simulink model "V3ASM"  (R2020b)
(part 2 of 23)

  Revolute39 : sm_lib/Joints/Revolute Joint  JointMode=Normal  SenseConstraintForce=off  SenseConstraintForceX=off  SenseConstraintForceY=off  SenseConstraintForceZ=off  SenseConstraintTorque=off  SenseConstraintTorqueX=off  SenseConstraintTorqueY=off  SenseConstraintTorqueZ=off  SenseTotalForce=off  SenseTotalForceX=off  SenseTotalForceY=off  SenseTotalForceZ=off  SenseTotalTorque=off  SenseTotalTorqueX=off  SenseTotalTorqueY=off  SenseTotalTorqueZ=off  CompositeWrenchDir=FollowerOnBase  CompositeWrenchFrame=BaseFrame  EquilibriumPosition=0  EquilibriumPositionUnits=deg  SpringStiffness=0  SpringStiffnessUnits=N*m/deg  DampingCoefficient=0  DampingCoefficientUnits=N*m/(deg/s)  TorqueActuationMode=NoTorque  MotionActuationMode=ComputedMotion  SensePosition=off  SenseVelocity=off  SenseAcceleration=off  SenseTorqueForce=off  SenseLowerLimitTorqueForce=off  SenseUpperLimitTorqueForce=off  LowerLimitSpecify=off  LowerLimitBound=-90  LowerLimitBoundUnits=deg  LowerLimitStiffness=1e4  LowerLimitStiffnessUnits=N*m/deg  LowerLimitDamping=10  LowerLimitDampingUnits=N*m/(deg/s)  LowerLimitTransitionRegionWidth=0.1  LowerLimitTransitionRegionWidthUnits=deg  UpperLimitSpecify=off  UpperLimitBound=90  UpperLimitBoundUnits=deg  UpperLimitStiffness=1e4  UpperLimitStiffnessUnits=N*m/deg  UpperLimitDamping=10  UpperLimitDampingUnits=N*m/(deg/s)  UpperLimitTransitionRegionWidth=0.1  UpperLimitTransitionRegionWidthUnits=deg  PositionTargetSpecify=on  PositionTargetPriority=Low  PositionTargetValue=smiData.RevoluteJoint(40).Rz.Pos  PositionTargetValueUnits=deg  VelocityTargetSpecify=off  VelocityTargetPriority=High  VelocityTargetValue=0  VelocityTargetValueUnits=deg/s
  Revolute4 : sm_lib/Joints/Revolute Joint  JointMode=Normal  SenseConstraintForce=off  SenseConstraintForceX=off  SenseConstraintForceY=off  SenseConstraintForceZ=off  SenseConstraintTorque=off  SenseConstraintTorqueX=off  SenseConstraintTorqueY=off  SenseConstraintTorqueZ=off  SenseTotalForce=off  SenseTotalForceX=off  SenseTotalForceY=off  SenseTotalForceZ=off  SenseTotalTorque=off  SenseTotalTorqueX=off  SenseTotalTorqueY=off  SenseTotalTorqueZ=off  CompositeWrenchDir=FollowerOnBase  CompositeWrenchFrame=BaseFrame  EquilibriumPosition=0  EquilibriumPositionUnits=deg  SpringStiffness=0  SpringStiffnessUnits=N*m/deg  DampingCoefficient=0  DampingCoefficientUnits=N*m/(deg/s)  TorqueActuationMode=NoTorque  MotionActuationMode=ComputedMotion  SensePosition=off  SenseVelocity=off  SenseAcceleration=off  SenseTorqueForce=off  SenseLowerLimitTorqueForce=off  SenseUpperLimitTorqueForce=off  LowerLimitSpecify=off  LowerLimitBound=-90  LowerLimitBoundUnits=deg  LowerLimitStiffness=1e4  LowerLimitStiffnessUnits=N*m/deg  LowerLimitDamping=10  LowerLimitDampingUnits=N*m/(deg/s)  LowerLimitTransitionRegionWidth=0.1  LowerLimitTransitionRegionWidthUnits=deg  UpperLimitSpecify=off  UpperLimitBound=90  UpperLimitBoundUnits=deg  UpperLimitStiffness=1e4  UpperLimitStiffnessUnits=N*m/deg  UpperLimitDamping=10  UpperLimitDampingUnits=N*m/(deg/s)  UpperLimitTransitionRegionWidth=0.1  UpperLimitTransitionRegionWidthUnits=deg  PositionTargetSpecify=on  PositionTargetPriority=Low  PositionTargetValue=smiData.RevoluteJoint(5).Rz.Pos  PositionTargetValueUnits=deg  VelocityTargetSpecify=off  VelocityTargetPriority=High  VelocityTargetValue=0  VelocityTargetValueUnits=deg/s
  Revolute40 : sm_lib/Joints/Revolute Joint  JointMode=Normal  SenseConstraintForce=off  SenseConstraintForceX=off  SenseConstraintForceY=off  SenseConstraintForceZ=off  SenseConstraintTorque=off  SenseConstraintTorqueX=off  SenseConstraintTorqueY=off  SenseConstraintTorqueZ=off  SenseTotalForce=off  SenseTotalForceX=off  SenseTotalForceY=off  SenseTotalForceZ=off  SenseTotalTorque=off  SenseTotalTorqueX=off  SenseTotalTorqueY=off  SenseTotalTorqueZ=off  CompositeWrenchDir=FollowerOnBase  CompositeWrenchFrame=BaseFrame  EquilibriumPosition=0  EquilibriumPositionUnits=deg  SpringStiffness=0  SpringStiffnessUnits=N*m/deg  DampingCoefficient=0  DampingCoefficientUnits=N*m/(deg/s)  TorqueActuationMode=NoTorque  MotionActuationMode=ComputedMotion  SensePosition=off  SenseVelocity=off  SenseAcceleration=off  SenseTorqueForce=off  SenseLowerLimitTorqueForce=off  SenseUpperLimitTorqueForce=off  LowerLimitSpecify=off  LowerLimitBound=-90  LowerLimitBoundUnits=deg  LowerLimitStiffness=1e4  LowerLimitStiffnessUnits=N*m/deg  LowerLimitDamping=10  LowerLimitDampingUnits=N*m/(deg/s)  LowerLimitTransitionRegionWidth=0.1  LowerLimitTransitionRegionWidthUnits=deg  UpperLimitSpecify=off  UpperLimitBound=90  UpperLimitBoundUnits=deg  UpperLimitStiffness=1e4  UpperLimitStiffnessUnits=N*m/deg  UpperLimitDamping=10  UpperLimitDampingUnits=N*m/(deg/s)  UpperLimitTransitionRegionWidth=0.1  UpperLimitTransitionRegionWidthUnits=deg  PositionTargetSpecify=on  PositionTargetPriority=Low  PositionTargetValue=smiData.RevoluteJoint(41).Rz.Pos  PositionTargetValueUnits=deg  VelocityTargetSpecify=off  VelocityTargetPriority=High  VelocityTargetValue=0  VelocityTargetValueUnits=deg/s
  Revolute41 : sm_lib/Joints/Revolute Joint  JointMode=Normal  SenseConstraintForce=off  SenseConstraintForceX=off  SenseConstraintForceY=off  SenseConstraintForceZ=off  SenseConstraintTorque=off  SenseConstraintTorqueX=off  SenseConstraintTorqueY=off  SenseConstraintTorqueZ=off  SenseTotalForce=off  SenseTotalForceX=off  SenseTotalForceY=off  SenseTotalForceZ=off  SenseTotalTorque=off  SenseTotalTorqueX=off  SenseTotalTorqueY=off  SenseTotalTorqueZ=off  CompositeWrenchDir=FollowerOnBase  CompositeWrenchFrame=BaseFrame  EquilibriumPosition=0  EquilibriumPositionUnits=deg  SpringStiffness=0  SpringStiffnessUnits=N*m/deg  DampingCoefficient=0  DampingCoefficientUnits=N*m/(deg/s)  TorqueActuationMode=NoTorque  MotionActuationMode=ComputedMotion  SensePosition=off  SenseVelocity=off  SenseAcceleration=off  SenseTorqueForce=off  SenseLowerLimitTorqueForce=off  SenseUpperLimitTorqueForce=off  LowerLimitSpecify=off  LowerLimitBound=-90  LowerLimitBoundUnits=deg  LowerLimitStiffness=1e4  LowerLimitStiffnessUnits=N*m/deg  LowerLimitDamping=10  LowerLimitDampingUnits=N*m/(deg/s)  LowerLimitTransitionRegionWidth=0.1  LowerLimitTransitionRegionWidthUnits=deg  UpperLimitSpecify=off  UpperLimitBound=90  UpperLimitBoundUnits=deg  UpperLimitStiffness=1e4  UpperLimitStiffnessUnits=N*m/deg  UpperLimitDamping=10  UpperLimitDampingUnits=N*m/(deg/s)  UpperLimitTransitionRegionWidth=0.1  UpperLimitTransitionRegionWidthUnits=deg  PositionTargetSpecify=on  PositionTargetPriority=Low  PositionTargetValue=smiData.RevoluteJoint(42).Rz.Pos  PositionTargetValueUnits=deg  VelocityTargetSpecify=off  VelocityTargetPriority=High  VelocityTargetValue=0  VelocityTargetValueUnits=deg/s
  Revolute5 : sm_lib/Joints/Revolute Joint  JointMode=Normal  SenseConstraintForce=off  SenseConstraintForceX=off  SenseConstraintForceY=off  SenseConstraintForceZ=off  SenseConstraintTorque=off  SenseConstraintTorqueX=off  SenseConstraintTorqueY=off  SenseConstraintTorqueZ=off  SenseTotalForce=off  SenseTotalForceX=off  SenseTotalForceY=off  SenseTotalForceZ=off  SenseTotalTorque=off  SenseTotalTorqueX=off  SenseTotalTorqueY=off  SenseTotalTorqueZ=off  CompositeWrenchDir=FollowerOnBase  CompositeWrenchFrame=BaseFrame  EquilibriumPosition=0  EquilibriumPositionUnits=deg  SpringStiffness=0  SpringStiffnessUnits=N*m/deg  DampingCoefficient=0  DampingCoefficientUnits=N*m/(deg/s)  TorqueActuationMode=NoTorque  MotionActuationMode=ComputedMotion  SensePosition=off  SenseVelocity=off  SenseAcceleration=off  SenseTorqueForce=off  SenseLowerLimitTorqueForce=off  SenseUpperLimitTorqueForce=off  LowerLimitSpecify=off  LowerLimitBound=-90  LowerLimitBoundUnits=deg  LowerLimitStiffness=1e4  LowerLimitStiffnessUnits=N*m/deg  LowerLimitDamping=10  LowerLimitDampingUnits=N*m/(deg/s)  LowerLimitTransitionRegionWidth=0.1  LowerLimitTransitionRegionWidthUnits=deg  UpperLimitSpecify=off  UpperLimitBound=90  UpperLimitBoundUnits=deg  UpperLimitStiffness=1e4  UpperLimitStiffnessUnits=N*m/deg  UpperLimitDamping=10  UpperLimitDampingUnits=N*m/(deg/s)  UpperLimitTransitionRegionWidth=0.1  UpperLimitTransitionRegionWidthUnits=deg  PositionTargetSpecify=on  PositionTargetPriority=Low  PositionTargetValue=smiData.RevoluteJoint(6).Rz.Pos  PositionTargetValueUnits=deg  VelocityTargetSpecify=off  VelocityTargetPriority=High  VelocityTargetValue=0  VelocityTargetValueUnits=deg/s
  Revolute6 : sm_lib/Joints/Revolute Joint  JointMode=Normal  SenseConstraintForce=off  SenseConstraintForceX=off  SenseConstraintForceY=off  SenseConstraintForceZ=off  SenseConstraintTorque=off  SenseConstraintTorqueX=off  SenseConstraintTorqueY=off  SenseConstraintTorqueZ=off  SenseTotalForce=off  SenseTotalForceX=off  SenseTotalForceY=off  SenseTotalForceZ=off  SenseTotalTorque=off  SenseTotalTorqueX=off  SenseTotalTorqueY=off  SenseTotalTorqueZ=off  CompositeWrenchDir=FollowerOnBase  CompositeWrenchFrame=BaseFrame  EquilibriumPosition=0  EquilibriumPositionUnits=deg  SpringStiffness=0  SpringStiffnessUnits=N*m/deg  DampingCoefficient=0  DampingCoefficientUnits=N*m/(deg/s)  TorqueActuationMode=NoTorque  MotionActuationMode=ComputedMotion  SensePosition=off  SenseVelocity=off  SenseAcceleration=off  SenseTorqueForce=off  SenseLowerLimitTorqueForce=off  SenseUpperLimitTorqueForce=off  LowerLimitSpecify=off  LowerLimitBound=-90  LowerLimitBoundUnits=deg  LowerLimitStiffness=1e4  LowerLimitStiffnessUnits=N*m/deg  LowerLimitDamping=10  LowerLimitDampingUnits=N*m/(deg/s)  LowerLimitTransitionRegionWidth=0.1  LowerLimitTransitionRegionWidthUnits=deg  UpperLimitSpecify=off  UpperLimitBound=90  UpperLimitBoundUnits=deg  UpperLimitStiffness=1e4  UpperLimitStiffnessUnits=N*m/deg  UpperLimitDamping=10  UpperLimitDampingUnits=N*m/(deg/s)  UpperLimitTransitionRegionWidth=0.1  UpperLimitTransitionRegionWidthUnits=deg  PositionTargetSpecify=on  PositionTargetPriority=Low  PositionTargetValue=smiData.RevoluteJoint(7).Rz.Pos  PositionTargetValueUnits=deg  VelocityTargetSpecify=off  VelocityTargetPriority=High  VelocityTargetValue=0  VelocityTargetValueUnits=deg/s
  Revolute7 : sm_lib/Joints/Revolute Joint  JointMode=Normal  SenseConstraintForce=off  SenseConstraintForceX=off  SenseConstraintForceY=off  SenseConstraintForceZ=off  SenseConstraintTorque=off  SenseConstraintTorqueX=off  SenseConstraintTorqueY=off  SenseConstraintTorqueZ=off  SenseTotalForce=off  SenseTotalForceX=off  SenseTotalForceY=off  SenseTotalForceZ=off  SenseTotalTorque=off  SenseTotalTorqueX=off  SenseTotalTorqueY=off  SenseTotalTorqueZ=off  CompositeWrenchDir=FollowerOnBase  CompositeWrenchFrame=BaseFrame  EquilibriumPosition=0  EquilibriumPositionUnits=deg  SpringStiffness=0  SpringStiffnessUnits=N*m/deg  DampingCoefficient=0  DampingCoefficientUnits=N*m/(deg/s)  TorqueActuationMode=NoTorque  MotionActuationMode=ComputedMotion  SensePosition=off  SenseVelocity=off  SenseAcceleration=off  SenseTorqueForce=off  SenseLowerLimitTorqueForce=off  SenseUpperLimitTorqueForce=off  LowerLimitSpecify=off  LowerLimitBound=-90  LowerLimitBoundUnits=deg  LowerLimitStiffness=1e4  LowerLimitStiffnessUnits=N*m/deg  LowerLimitDamping=10  LowerLimitDampingUnits=N*m/(deg/s)  LowerLimitTransitionRegionWidth=0.1  LowerLimitTransitionRegionWidthUnits=deg  UpperLimitSpecify=off  UpperLimitBound=90  UpperLimitBoundUnits=deg  UpperLimitStiffness=1e4  UpperLimitStiffnessUnits=N*m/deg  UpperLimitDamping=10  UpperLimitDampingUnits=N*m/(deg/s)  UpperLimitTransitionRegionWidth=0.1  UpperLimitTransitionRegionWidthUnits=deg  PositionTargetSpecify=on  PositionTargetPriority=Low  PositionTargetValue=smiData.RevoluteJoint(8).Rz.Pos  PositionTargetValueUnits=deg  VelocityTargetSpecify=off  VelocityTargetPriority=High  VelocityTargetValue=0  VelocityTargetValueUnits=deg/s
  Revolute8 : sm_lib/Joints/Revolute Joint  JointMode=Normal  SenseConstraintForce=off  SenseConstraintForceX=off  SenseConstraintForceY=off  SenseConstraintForceZ=off  SenseConstraintTorque=off  SenseConstraintTorqueX=off  SenseConstraintTorqueY=off  SenseConstraintTorqueZ=off  SenseTotalForce=off  SenseTotalForceX=off  SenseTotalForceY=off  SenseTotalForceZ=off  SenseTotalTorque=off  SenseTotalTorqueX=off  SenseTotalTorqueY=off  SenseTotalTorqueZ=off  CompositeWrenchDir=FollowerOnBase  CompositeWrenchFrame=BaseFrame  EquilibriumPosition=0  EquilibriumPositionUnits=deg  SpringStiffness=0  SpringStiffnessUnits=N*m/deg  DampingCoefficient=0  DampingCoefficientUnits=N*m/(deg/s)  TorqueActuationMode=NoTorque  MotionActuationMode=ComputedMotion  SensePosition=off  SenseVelocity=off  SenseAcceleration=off  SenseTorqueForce=off  SenseLowerLimitTorqueForce=off  SenseUpperLimitTorqueForce=off  LowerLimitSpecify=off  LowerLimitBound=-90  LowerLimitBoundUnits=deg  LowerLimitStiffness=1e4  LowerLimitStiffnessUnits=N*m/deg  LowerLimitDamping=10  LowerLimitDampingUnits=N*m/(deg/s)  LowerLimitTransitionRegionWidth=0.1  LowerLimitTransitionRegionWidthUnits=deg  UpperLimitSpecify=off  UpperLimitBound=90  UpperLimitBoundUnits=deg  UpperLimitStiffness=1e4  UpperLimitStiffnessUnits=N*m/deg  UpperLimitDamping=10  UpperLimitDampingUnits=N*m/(deg/s)  UpperLimitTransitionRegionWidth=0.1  UpperLimitTransitionRegionWidthUnits=deg  PositionTargetSpecify=on  PositionTargetPriority=Low  PositionTargetValue=smiData.RevoluteJoint(9).Rz.Pos  PositionTargetValueUnits=deg  VelocityTargetSpecify=off  VelocityTargetPriority=High  VelocityTargetValue=0  VelocityTargetValueUnits=deg/s
  Revolute9 : sm_lib/Joints/Revolute Joint  JointMode=Normal  SenseConstraintForce=off  SenseConstraintForceX=off  SenseConstraintForceY=off  SenseConstraintForceZ=off  SenseConstraintTorque=off  SenseConstraintTorqueX=off  SenseConstraintTorqueY=off  SenseConstraintTorqueZ=off  SenseTotalForce=off  SenseTotalForceX=off  SenseTotalForceY=off  SenseTotalForceZ=off  SenseTotalTorque=off  SenseTotalTorqueX=off  SenseTotalTorqueY=off  SenseTotalTorqueZ=off  CompositeWrenchDir=FollowerOnBase  CompositeWrenchFrame=BaseFrame  EquilibriumPosition=0  EquilibriumPositionUnits=deg  SpringStiffness=0  SpringStiffnessUnits=N*m/deg  DampingCoefficient=0  DampingCoefficientUnits=N*m/(deg/s)  TorqueActuationMode=NoTorque  MotionActuationMode=ComputedMotion  SensePosition=off  SenseVelocity=off  SenseAcceleration=off  SenseTorqueForce=off  SenseLowerLimitTorqueForce=off  SenseUpperLimitTorqueForce=off  LowerLimitSpecify=off  LowerLimitBound=-90  LowerLimitBoundUnits=deg  LowerLimitStiffness=1e4  LowerLimitStiffnessUnits=N*m/deg  LowerLimitDamping=10  LowerLimitDampingUnits=N*m/(deg/s)  LowerLimitTransitionRegionWidth=0.1  LowerLimitTransitionRegionWidthUnits=deg  UpperLimitSpecify=off  UpperLimitBound=90  UpperLimitBoundUnits=deg  UpperLimitStiffness=1e4  UpperLimitStiffnessUnits=N*m/deg  UpperLimitDamping=10  UpperLimitDampingUnits=N*m/(deg/s)  UpperLimitTransitionRegionWidth=0.1  UpperLimitTransitionRegionWidthUnits=deg  PositionTargetSpecify=on  PositionTargetPriority=Low  PositionTargetValue=smiData.RevoluteJoint(10).Rz.Pos  PositionTargetValueUnits=deg  VelocityTargetSpecify=off  VelocityTargetPriority=High  VelocityTargetValue=0  VelocityTargetValueUnits=deg/s
  Right_Femur_1_RIGID : Subsystem
  Right_Femur_2_RIGID : Subsystem
  Right_Femur_3_RIGID : Subsystem
      settings: PortSchema="{\"entries\":[{\"content\":{\"sides\":[{\"content\":{\"connectorIds\":[\"LConn1\",\"LConn2\"]},\"type\":\"ConnectorPlacement.EquallySpacedRectSide\",\"uuid\":\"6e9f23bc-e754-4da4-8930-138de5532f90\"},{\"content\":{\"connectorIds\":[\"RConn1\",\"RConn2\"],\"side\":\"RIGHT\"},\"type\":\"ConnectorPlacement.EquallySpacedRectSide\",\"uuid\":\"91478b6a-22d5-43c7-a35d-28ad478b6bd6\"},{\"content\":{\"connectorIds\":[],\"side\":\"TOP\"},\"type\":\"ConnectorPlacement.EquallySpacedRectSide\",\"uuid\":\"a1bbb7f2-676b-4a5f-8f1f-94155cb0c297\"},{\"content\":{\"connectorIds\":[\"RConn3\"],\"side\":\"BOTTOM\"},\"type\":\"ConnectorPlacement.EquallySpacedRectSide\",\"uuid\":\"a740551b-024f-4afc-80fa-8619e7f29db2\"},{\"content\":{\"connectorIds\":[],\"side\":\"HIDDEN\"},\"type\":\"ConnectorPlacement.EquallySpacedRectSide\",\"uuid\":\"6117f7a1-a6d4-4a0b-8d67-f4151c91f03b\"}]},\"type\":\"ConnectorPlacement.EquallySpacedConnector\",\"uuid\":\"88f38e2e-088a-40bc-b46a-3a636d5d8d91\"}],\"packageUris\":[\"http://schema.mathworks.com/mf0/Connector/R2020b\"],\"version\":\"1.0\"}"
  Right_Tibia_1_RIGID : Subsystem
      settings: PortSchema="{\"entries\":[{\"content\":{\"sides\":[{\"content\":{\"connectorIds\":[]},\"type\":\"ConnectorPlacement.EquallySpacedRectSide\",\"uuid\":\"074441a8-d9e4-487c-8c33-9b67e272a773\"},{\"content\":{\"connectorIds\":[],\"side\":\"RIGHT\"},\"type\":\"ConnectorPlacement.EquallySpacedRectSide\",\"uuid\":\"1e1e3420-14cc-4c55-82ab-a2e10ec9c363\"},{\"content\":{\"connectorIds\":[\"LConn1\"],\"side\":\"TOP\"},\"type\":\"ConnectorPlacement.EquallySpacedRectSide\",\"uuid\":\"ee3632b0-5789-432c-9fdd-f21da32c2c6f\"},{\"content\":{\"connectorIds\":[\"RConn1\"],\"side\":\"BOTTOM\"},\"type\":\"ConnectorPlacement.EquallySpacedRectSide\",\"uuid\":\"6a666aa6-ddd6-4820-8f74-1465942c9f53\"},{\"content\":{\"connectorIds\":[],\"side\":\"HIDDEN\"},\"type\":\"ConnectorPlacement.EquallySpacedRectSide\",\"uuid\":\"c90d3278-8761-4bcd-83d9-2ae8a1d3adea\"}]},\"type\":\"ConnectorPlacement.EquallySpacedConnector\",\"uuid\":\"5e95a6d1-4844-49ea-8110-dc837ef3fc27\"}],\"packageUris\":[\"http://schema.mathworks.com/mf0/Connector/R2020b\"],\"version\":\"1.0\"}"
  Right_Tibia_2_RIGID : Subsystem
      settings: PortSchema="{\"entries\":[{\"content\":{\"sides\":[{\"content\":{\"connectorIds\":[]},\"type\":\"ConnectorPlacement.EquallySpacedRectSide\",\"uuid\":\"074441a8-d9e4-487c-8c33-9b67e272a773\"},{\"content\":{\"connectorIds\":[],\"side\":\"RIGHT\"},\"type\":\"ConnectorPlacement.EquallySpacedRectSide\",\"uuid\":\"1e1e3420-14cc-4c55-82ab-a2e10ec9c363\"},{\"content\":{\"connectorIds\":[\"LConn1\"],\"side\":\"TOP\"},\"type\":\"ConnectorPlacement.EquallySpacedRectSide\",\"uuid\":\"ee3632b0-5789-432c-9fdd-f21da32c2c6f\"},{\"content\":{\"connectorIds\":[\"RConn1\"],\"side\":\"BOTTOM\"},\"type\":\"ConnectorPlacement.EquallySpacedRectSide\",\"uuid\":\"151a3216-a789-41f2-a185-6e4e3a5d0a71\"},{\"content\":{\"connectorIds\":[],\"side\":\"HIDDEN\"},\"type\":\"ConnectorPlacement.EquallySpacedRectSide\",\"uuid\":\"c90d3278-8761-4bcd-83d9-2ae8a1d3adea\"}]},\"type\":\"ConnectorPlacement.EquallySpacedConnector\",\"uuid\":\"5e95a6d1-4844-49ea-8110-dc837ef3fc27\"}],\"packageUris\":[\"http://schema.mathworks.com/mf0/Connector/R2020b\"],\"version\":\"1.0\"}"
  Right_Tibia_3_RIGID : Subsystem
  Servo_example_1_RIGID : Subsystem
  Solver Configuration : nesl_utility/Solver Configuration  PhysicalDomain=network_engine_domain  SubClassName=solver  LeftPortType=input  RightPortType=generic  Tones=[]  Harmonics=[]  SimulateNoise=off  Profile=off  UseLocalSampling=off  EnableSwitchedLinearOptims=on  FrequencyDomain=off  UseCCode=off  RelTol=0.001  AbsTol=1e-06  MinStep=1e-09  ToWorkspace=off  RevertToSquareIcSolve=off  NumHomotopyIterations=100  PhasorMode=off  PhasorModeNumHarmonics=1  DoDC=off  ResidualTolerance=1e-09  UseLocalSolver=off  LocalSolverChoice=NE_BACKWARD_EULER_ADVANCER  LocalSolverSampleTime=0.001  DoFixedCost=off  MaxNonlinIter=3  MaxModeIter=2  ComputeImpulses=off  ImpulseIterations=2  LinearAlgebra=auto  EquationFormulation=NE_TIME_EF  DelaysMemoryBudget=1024  AutomaticFiltering=on  FilteringTimeConstant=0.001  PartitionStorageMethod=AS_NEEDED  PartitionMemoryBudget=1024  PartitionMethod=ROBUST
  Thorax_1_RIGID : Subsystem
  Transform : sm_lib/Frames and Transforms/Rigid Transform  TranslationMethod=Cartesian  TranslationStandardOffset=0  TranslationLengthUnit=mm  TranslationStandardAxis=+Z  TranslationCartesianOffset=smiData.RigidTransform(650).translation  TranslationROffset=0  TranslationROffsetUnits=m  TranslationZOffset=0  TranslationZOffsetUnits=m  TranslationThetaOffset=0  TranslationThetaOffsetUnits=deg  RotationMethod=ArbitraryAxis  RotationAngleUnits=rad  RotationStandardAxis=+Z  RotationAngle=smiData.RigidTransform(650).angle  RotationArbitraryAxis=smiData.RigidTransform(650).axis  FollAlignAxisA=+X  BaseAlignAxisA=+Y  FollAlignAxisB=+Y  BaseAlignAxisB=+Z  RotationSequenceAxes=FollowerAxes  RotationSequence=XYX  RotationSequenceAngles=[0 0 0]  RotationSequenceAnglesUnits=deg  RotationMatrix=[1 0 0; 0 1 0; 0 0 1]
  World : sm_lib/Frames and Transforms/World Frame
  battery_cover_1_RIGID : Subsystem
  cover_1_RIGID : Subsystem
  tilt_component_1_RIGID : Subsystem
  x0_625_bearring_10_RIGID : Subsystem
  x0_625_bearring_11_RIGID : Subsystem
  x0_625_bearring_12_RIGID : Subsystem
  x0_625_bearring_13_RIGID : Subsystem
      settings: PortSchema="{\"entries\":[{\"content\":{\"sides\":[{\"content\":{\"connectorIds\":[]},\"type\":\"ConnectorPlacement.EquallySpacedRectSide\",\"uuid\":\"9b113eda-c964-4a40-a098-4848f4ec2a27\"},{\"content\":{\"connectorIds\":[],\"side\":\"RIGHT\"},\"type\":\"ConnectorPlacement.EquallySpacedRectSide\",\"uuid\":\"11ab73dd-ba87-4183-b88c-15097fc1ecc4\"},{\"content\":{\"connectorIds\":[\"LConn1\"],\"side\":\"TOP\"},\"type\":\"ConnectorPlacement.EquallySpacedRectSide\",\"uuid\":\"f4251f55-f86d-4e49-9279-bfee74799eea\"},{\"content\":{\"connectorIds\":[\"RConn1\"],\"side\":\"BOTTOM\"},\"type\":\"ConnectorPlacement.EquallySpacedRectSide\",\"uuid\":\"24c71ed4-8185-4c72-8aa9-fe0f005f91b5\"},{\"content\":{\"connectorIds\":[],\"side\":\"HIDDEN\"},\"type\":\"ConnectorPlacement.EquallySpacedRectSide\",\"uuid\":\"7d96a6b7-c7a1-4c13-b2a1-8a4d6ed421c4\"}]},\"type\":\"ConnectorPlacement.EquallySpacedConnector\",\"uuid\":\"c8d18577-beef-4b76-b049-f443fd37a4ee\"}],\"packageUris\":[\"http://schema.mathworks.com/mf0/Connector/R2020b\"],\"version\":\"1.0\"}"
  x0_625_bearring_14_RIGID : Subsystem
      settings: PortSchema="{\"entries\":[{\"content\":{\"sides\":[{\"content\":{\"connectorIds\":[]},\"type\":\"ConnectorPlacement.EquallySpacedRectSide\",\"uuid\":\"3da95752-8f98-417b-8295-61e524b00241\"},{\"content\":{\"connectorIds\":[],\"side\":\"RIGHT\"},\"type\":\"ConnectorPlacement.EquallySpacedRectSide\",\"uuid\":\"08920931-2b6a-41f4-b54d-f07f12994704\"},{\"content\":{\"connectorIds\":[\"LConn1\"],\"side\":\"TOP\"},\"type\":\"ConnectorPlacement.EquallySpacedRectSide\",\"uuid\":\"06060dd0-52f7-4ddb-8536-795a2a5c474f\"},{\"content\":{\"connectorIds\":[\"RConn1\"],\"side\":\"BOTTOM\"},\"type\":\"ConnectorPlacement.EquallySpacedRectSide\",\"uuid\":\"7d0f6cbe-5266-42ef-84ce-a915496abbe7\"},{\"content\":{\"connectorIds\":[],\"side\":\"HIDDEN\"},\"type\":\"ConnectorPlacement.EquallySpacedRectSide\",\"uuid\":\"ec4288d9-14fe-4d0a-aaef-a07b505a15cf\"}]},\"type\":\"ConnectorPlacement.EquallySpacedConnector\",\"uuid\":\"eef58f47-4645-4554-bc58-27a3ecdd85a9\"}],\"packageUris\":[\"http://schema.mathworks.com/mf0/Connector/R2020b\"],\"version\":\"1.0\"}"
  x0_625_bearring_15_RIGID : Subsystem
  x0_625_bearring_16_RIGID : Subsystem
  x0_625_bearring_17_RIGID : Subsystem
  x0_625_bearring_18_RIGID : Subsystem
  x0_625_bearring_19_RIGID : Subsystem
      settings: PortSchema="{\"entries\":[{\"content\":{\"sides\":[{\"content\":{\"connectorIds\":[]},\"type\":\"ConnectorPlacement.EquallySpacedRectSide\",\"uuid\":\"9b113eda-c964-4a40-a098-4848f4ec2a27\"},{\"content\":{\"connectorIds\":[\"RConn1\"],\"side\":\"RIGHT\"},\"type\":\"ConnectorPlacement.EquallySpacedRectSide\",\"uuid\":\"11ab73dd-ba87-4183-b88c-15097fc1ecc4\"},{\"content\":{\"connectorIds\":[],\"side\":\"TOP\"},\"type\":\"ConnectorPlacement.EquallySpacedRectSide\",\"uuid\":\"f4251f55-f86d-4e49-9279-bfee74799eea\"},{\"content\":{\"connectorIds\":[\"RConn2\"],\"side\":\"BOTTOM\"},\"type\":\"ConnectorPlacement.EquallySpacedRectSide\",\"uuid\":\"7490bac8-7faa-4601-ae51-db4d0795f4bb\"},{\"content\":{\"connectorIds\":[],\"side\":\"HIDDEN\"},\"type\":\"ConnectorPlacement.EquallySpacedRectSide\",\"uuid\":\"7d96a6b7-c7a1-4c13-b2a1-8a4d6ed421c4\"}]},\"type\":\"ConnectorPlacement.EquallySpacedConnector\",\"uuid\":\"c8d18577-beef-4b76-b049-f443fd37a4ee\"}],\"packageUris\":[\"http://schema.mathworks.com/mf0/Connector/R2020b\"],\"version\":\"1.0\"}"
  x0_625_bearring_1_RIGID : Subsystem
  x0_625_bearring_2_RIGID : Subsystem
  x0_625_bearring_3_RIGID : Subsystem
      settings: PortSchema="{\"entries\":[{\"content\":{\"sides\":[{\"content\":{\"connectorIds\":[\"LConn1\"]},\"type\":\"ConnectorPlacement.EquallySpacedRectSide\",\"uuid\":\"074441a8-d9e4-487c-8c33-9b67e272a773\"},{\"content\":{\"connectorIds\":[],\"side\":\"RIGHT\"},\"type\":\"ConnectorPlacement.EquallySpacedRectSide\",\"uuid\":\"1e1e3420-14cc-4c55-82ab-a2e10ec9c363\"},{\"content\":{\"connectorIds\":[],\"side\":\"TOP\"},\"type\":\"ConnectorPlacement.EquallySpacedRectSide\",\"uuid\":\"ee3632b0-5789-432c-9fdd-f21da32c2c6f\"},{\"content\":{\"connectorIds\":[\"RConn1\"],\"side\":\"BOTTOM\"},\"type\":\"ConnectorPlacement.EquallySpacedRectSide\",\"uuid\":\"9c10dca8-2282-480c-a709-2bf465a4722a\"},{\"content\":{\"connectorIds\":[],\"side\":\"HIDDEN\"},\"type\":\"ConnectorPlacement.EquallySpacedRectSide\",\"uuid\":\"c90d3278-8761-4bcd-83d9-2ae8a1d3adea\"}]},\"type\":\"ConnectorPlacement.EquallySpacedConnector\",\"uuid\":\"5e95a6d1-4844-49ea-8110-dc837ef3fc27\"}],\"packageUris\":[\"http://schema.mathworks.com/mf0/Connector/R2020b\"],\"version\":\"1.0\"}"
  x0_625_bearring_4_RIGID : Subsystem
      settings: PortSchema="{\"entries\":[{\"content\":{\"sides\":[{\"content\":{\"connectorIds\":[]},\"type\":\"ConnectorPlacement.EquallySpacedRectSide\",\"uuid\":\"9b113eda-c964-4a40-a098-4848f4ec2a27\"},{\"content\":{\"connectorIds\":[],\"side\":\"RIGHT\"},\"type\":\"ConnectorPlacement.EquallySpacedRectSide\",\"uuid\":\"11ab73dd-ba87-4183-b88c-15097fc1ecc4\"},{\"content\":{\"connectorIds\":[\"LConn1\"],\"side\":\"TOP\"},\"type\":\"ConnectorPlacement.EquallySpacedRectSide\",\"uuid\":\"f4251f55-f86d-4e49-9279-bfee74799eea\"},{\"content\":{\"connectorIds\":[\"RConn1\"],\"side\":\"BOTTOM\"},\"type\":\"ConnectorPlacement.EquallySpacedRectSide\",\"uuid\":\"98871714-32fb-4668-adb6-48a0dfde2f43\"},{\"content\":{\"connectorIds\":[],\"side\":\"HIDDEN\"},\"type\":\"ConnectorPlacement.EquallySpacedRectSide\",\"uuid\":\"7d96a6b7-c7a1-4c13-b2a1-8a4d6ed421c4\"}]},\"type\":\"ConnectorPlacement.EquallySpacedConnector\",\"uuid\":\"c8d18577-beef-4b76-b049-f443fd37a4ee\"}],\"packageUris\":[\"http://schema.mathworks.com/mf0/Connector/R2020b\"],\"version\":\"1.0\"}"
  x0_625_bearring_5_RIGID : Subsystem
  x0_625_bearring_6_RIGID : Subsystem
  x0_625_bearring_7_RIGID : Subsystem
  x0_625_bearring_8_RIGID : Subsystem
  x0_625_bearring_9_RIGID : Subsystem
  x12Channel_PWM_v1_1_RIGID : Subsystem
  x12Channel_PWM_v1_2_RIGID : Subsystem
  connections:
  MechanismConfiguration/RConn1 -- Transform/LConn1 -- Solver Configuration/RConn1 -- World/RConn1
  Coxa_9_RIGID/LConn1 -- Revolute/LConn1
  DS3218MG_v1_13_RIGID/LConn1 -- Revolute3/RConn1
  Revolute22/RConn1 -- x0_625_bearring_1_RIGID/LConn2
  Abdomen_1_RIGID/RConn8 -- Planar6/LConn1
  Planar6/RConn1 -- x0_625_bearring_3_RIGID/LConn1
  Coxa_12_RIGID/RConn1 -- Revolute23/LConn1
  Revolute23/RConn1 -- x0_625_bearring_4_RIGID/LConn1
  Revolute24/LConn1 -- x0_625_bearring_4_RIGID/RConn1
  Left_Femur_1_RIGID/RConn1 -- Revolute24/RConn1
  Coxa_13_RIGID/LConn2 -- Revolute25/LConn1
  Revolute25/RConn1 -- x0_625_bearring_5_RIGID/LConn1
  Cylindrical3/LConn1 -- x0_625_bearring_5_RIGID/RConn1
  DS3218MG_v1_13_RIGID/RConn1 -- Parallel1/LConn1
  Cylindrical3/RConn1 -- Left_Femur_2_RIGID/LConn1
  Abdomen_1_RIGID/RConn2 -- Planar7/LConn1
  Planar7/RConn1 -- x0_625_bearring_6_RIGID/LConn1
  Cylindrical4/LConn1 -- x0_625_bearring_7_RIGID/LConn1
  Cylindrical4/RConn1 -- Left_Femur_3_RIGID/LConn2
  Abdomen_1_RIGID/RConn1 -- Planar8/LConn1
  Planar8/RConn1 -- x0_625_bearring_8_RIGID/LConn1
  Prismatic1/LConn1 -- x12Channel_PWM_v1_1_RIGID/RConn1
  Prismatic1/RConn1 -- x12Channel_PWM_v1_2_RIGID/LConn2
  Coxa_10_RIGID/RConn2 -- Revolute26/LConn1
  Left_Femur_2_RIGID/LConn3 -- Parallel1/RConn1
  DS3218MG_v1_9_RIGID/LConn1 -- Revolute26/RConn1
  Coxa_13_RIGID/RConn1 -- Planar9/LConn1
  Left_Femur_2_RIGID/LConn2 -- Planar9/RConn1
  Abdomen_1_RIGID/LConn7 -- DS3218MG_v1_1_RIGID/LConn2
  Abdomen_1_RIGID/LConn6 -- DS3218MG_v1_4_RIGID/LConn1
  Abdomen_1_RIGID/LConn5 -- DS3218MG_v1_5_RIGID/LConn1
  Abdomen_1_RIGID/LConn4 -- DS3218MG_v1_6_RIGID/LConn1
  DS3218MG_v1_7_RIGID/LConn2 -- Pan_component_1_RIGID/LConn1
  Cylindrical5/LConn1 -- Pan_component_1_RIGID/RConn1
  Cylindrical5/RConn1 -- DS3218MG_v1_8_RIGID/LConn2
  Coxa_12_RIGID/LConn2 -- Revolute4/LConn1
  Servo_example_1_RIGID/LConn1 -- Thorax_1_RIGID/LConn4
  Revolute27/LConn1 -- Servo_example_1_RIGID/RConn1
  Abdomen_1_RIGID/LConn3 -- Revolute27/RConn1
  Abdomen_1_RIGID/LConn2 -- Jetson_nano_fixed_v1_1_RIGID/LConn3
  Cover_Abdomen_1_RIGID/RConn2 -- Prismatic2/LConn1
  Prismatic2/RConn1 -- x12Channel_PWM_v1_1_RIGID/LConn1
  Cover_Abdomen_1_RIGID/RConn1 -- Revolute28/LConn1
  Revolute28/RConn1 -- x12Channel_PWM_v1_2_RIGID/LConn1
  Abdomen_1_RIGID/LConn1 -- Cover_Abdomen_1_RIGID/LConn3
  Adafruit_BNO055_AP214_v1_1_RIGID/LConn1 -- Cover_Abdomen_1_RIGID/LConn2
  DS3218MG_v1_14_RIGID/LConn1 -- Revolute4/RConn1
  Cover_Abdomen_1_RIGID/LConn1 -- cover_1_RIGID/LConn1
  Revolute29/LConn1 -- Thorax_1_RIGID/RConn1
  Cap_1_RIGID/LConn1 -- Revolute29/RConn1
  Cap_1_RIGID/RConn1 -- Cylindrical6/LConn1
  Cylindrical6/RConn1 -- x0_625_bearring_12_RIGID/LConn2
  Abdomen_1_RIGID/RConn7 -- Revolute30/LConn1
  Cap_2_RIGID/LConn1 -- Revolute30/RConn1
  Cap_2_RIGID/RConn1 -- Cylindrical7/LConn1
  Cylindrical7/RConn1 -- x0_625_bearring_10_RIGID/LConn2
  Cap_3_RIGID/RConn1 -- Cylindrical8/LConn1
  DS3218MG_v1_14_RIGID/RConn1 -- Parallel2/LConn1
  Cylindrical8/RConn1 -- x0_625_bearring_8_RIGID/LConn2
  Abdomen_1_RIGID/RConn6 -- Revolute31/LConn1
  Cap_3_RIGID/LConn1 -- Revolute31/RConn1
  Revolute32/LConn1 -- Thorax_1_RIGID/RConn3
  Cap_4_RIGID/LConn1 -- Revolute32/RConn1
  Cap_4_RIGID/RConn1 -- Cylindrical9/LConn1
  Cylindrical9/RConn1 -- x0_625_bearring_2_RIGID/LConn1
  Cap_5_RIGID/RConn1 -- Cylindrical10/LConn1
  Cylindrical10/RConn1 -- x0_625_bearring_3_RIGID/RConn1
  Abdomen_1_RIGID/RConn5 -- Revolute33/LConn1
  Left_Femur_1_RIGID/LConn1 -- Parallel2/RConn1
  Cap_5_RIGID/LConn1 -- Revolute33/RConn1
  Cap_6_RIGID/RConn1 -- Cylindrical11/LConn1
  Cylindrical11/RConn1 -- x0_625_bearring_6_RIGID/LConn2
  Abdomen_1_RIGID/RConn4 -- Revolute34/LConn1
  Cap_6_RIGID/RConn2 -- Revolute34/RConn1
  IntelRealsense_D435_Multibody_1_RIGID/LConn1 -- tilt_component_1_RIGID/LConn2
  Revolute35/LConn1 -- tilt_component_1_RIGID/RConn2
  Revolute35/RConn1 -- x0_625_bearring_1_RIGID/LConn1
  Intel_RealSense_T265_1_1_RIGID/LConn1 -- tilt_component_1_RIGID/LConn1
  Planar10/LConn1 -- tilt_component_1_RIGID/RConn1
  DS3218MG_v1_15_RIGID/RConn1 -- Rectangular/LConn1
  DS3218MG_v1_8_RIGID/LConn1 -- Planar10/RConn1
  Abdomen_1_RIGID/RConn3 -- Planar11/LConn1
  Planar11/RConn1 -- x0_625_bearring_10_RIGID/LConn1
  Coxa_10_RIGID/LConn2 -- Revolute36/LConn1
  Revolute36/RConn1 -- x0_625_bearring_11_RIGID/LConn1
  Planar12/LConn1 -- Thorax_1_RIGID/LConn1
  Planar12/RConn1 -- x0_625_bearring_12_RIGID/LConn1
  Coxa_11_RIGID/LConn1 -- Revolute37/LConn1
  Revolute37/RConn1 -- x0_625_bearring_13_RIGID/LConn1
  Cylindrical12/LConn1 -- x0_625_bearring_14_RIGID/RConn1
  Left_Tibia_1_RIGID/LConn1 -- Rectangular/RConn1
  Cylindrical12/RConn1 -- Left_Tibia_1_RIGID/RConn1
  Revolute38/LConn1 -- x0_625_bearring_14_RIGID/LConn1
  Left_Femur_1_RIGID/RConn2 -- Revolute38/RConn1
  Cylindrical13/LConn1 -- x0_625_bearring_15_RIGID/RConn1
  Cylindrical13/RConn1 -- Left_Tibia_2_RIGID/LConn1
  Revolute39/LConn1 -- x0_625_bearring_15_RIGID/LConn1
  Left_Femur_2_RIGID/LConn4 -- Revolute39/RConn1
  Cylindrical14/LConn1 -- x0_625_bearring_16_RIGID/RConn1
  Cylindrical14/RConn1 -- Left_Tibia_3_RIGID/LConn1
  Revolute40/LConn1 -- x0_625_bearring_16_RIGID/RConn2
  DS3218MG_v1_15_RIGID/LConn1 -- Revolute5/LConn1
  Left_Femur_3_RIGID/LConn1 -- Revolute40/RConn1
  Cylindrical15/LConn1 -- x0_625_bearring_17_RIGID/RConn1
  Cylindrical15/RConn1 -- Right_Tibia_3_RIGID/RConn1
  Cylindrical16/LConn1 -- x0_625_bearring_18_RIGID/RConn1
  Cylindrical16/RConn1 -- Right_Tibia_2_RIGID/LConn1
  Cylindrical17/LConn1 -- x0_625_bearring_19_RIGID/RConn2
  Cylindrical17/RConn1 -- Right_Tibia_1_RIGID/LConn1
  Jetson_nano_fixed_v1_1_RIGID/LConn2 -- Noctua_Fan_NF_A4x10_40mm_v1_1_RIGID/LConn1
  Ankor_1_RIGID/LConn1 -- Cover_Thorax_1_RIGID/LConn2
  Ankor_1_RIGID/RConn1 -- Revolute41/LConn1
  DS3218MG_v1_10_RIGID/RConn1 -- Revolute/RConn1
  Left_Femur_1_RIGID/LConn2 -- Revolute5/RConn1
  DS3218MG_v1_7_RIGID/LConn1 -- Revolute41/RConn1
  Jetson_nano_fixed_v1_1_RIGID/LConn1 -- Transform/RConn1
  DS3218MG_v1_16_RIGID/LConn1 -- Rectangular1/LConn1
  Left_Tibia_2_RIGID/RConn1 -- Rectangular1/RConn1
  DS3218MG_v1_16_RIGID/RConn1 -- Revolute6/LConn1
  Left_Femur_2_RIGID/RConn1 -- Revolute6/RConn1
  DS3218MG_v1_17_RIGID/RConn1 -- Rectangular2/LConn1
  Left_Tibia_3_RIGID/RConn1 -- Rectangular2/RConn1
  DS3218MG_v1_17_RIGID/RConn2 -- Revolute7/LConn1
  Left_Femur_3_RIGID/RConn1 -- Revolute7/RConn1
  DS3218MG_v1_18_RIGID/RConn1 -- Rectangular3/LConn1
  Coxa_11_RIGID/RConn2 -- Revolute1/LConn1
  Rectangular3/RConn1 -- Right_Tibia_3_RIGID/LConn1
  DS3218MG_v1_19_RIGID/RConn1 -- Rectangular4/LConn1
  Rectangular4/RConn1 -- Right_Tibia_2_RIGID/RConn1
  DS3218MG_v1_20_RIGID/RConn1 -- Rectangular5/LConn1
  Rectangular5/RConn1 -- Right_Tibia_1_RIGID/RConn1
  Revolute8/LConn1 -- Right_Femur_1_RIGID/LConn2
  DS3218MG_v1_19_RIGID/LConn1 -- Revolute8/RConn1
  Coxa_10_RIGID/LConn1 -- Planar/LConn1
  Planar/RConn1 -- Right_Femur_1_RIGID/RConn2
  DS3218MG_v1_9_RIGID/RConn1 -- Parallel3/LConn1
  DS3218MG_v1_11_RIGID/LConn1 -- Revolute1/RConn1
  Parallel3/RConn1 -- Right_Femur_1_RIGID/RConn3
  Cylindrical/LConn1 -- x0_625_bearring_11_RIGID/RConn1
  Cylindrical/RConn1 -- Right_Femur_1_RIGID/RConn1
  Revolute9/LConn1 -- Right_Femur_1_RIGID/LConn1
  Revolute9/RConn1 -- x0_625_bearring_18_RIGID/LConn1
  DS3218MG_v1_11_RIGID/RConn1 -- Parallel4/LConn1
  Parallel4/RConn1 -- Right_Femur_2_RIGID/RConn1
  Revolute10/LConn1 -- Right_Femur_2_RIGID/RConn2
  DS3218MG_v1_20_RIGID/LConn1 -- Revolute10/RConn1
  Coxa_11_RIGID/RConn1 -- Planar1/LConn1
  Coxa_8_RIGID/RConn1 -- Revolute2/LConn1
  Planar1/RConn1 -- Right_Femur_2_RIGID/LConn2
  Cylindrical1/LConn1 -- x0_625_bearring_13_RIGID/RConn1
  Cylindrical1/RConn1 -- Right_Femur_2_RIGID/LConn1
  Revolute11/LConn1 -- Right_Femur_2_RIGID/LConn3
  Revolute11/RConn1 -- x0_625_bearring_19_RIGID/RConn1
  DS3218MG_v1_10_RIGID/LConn1 -- Parallel5/LConn1
  Parallel5/RConn1 -- Right_Femur_3_RIGID/LConn2
  Revolute12/LConn1 -- Right_Femur_3_RIGID/LConn1
  DS3218MG_v1_18_RIGID/LConn1 -- Revolute12/RConn1
  Coxa_9_RIGID/LConn2 -- Planar2/LConn1
  DS3218MG_v1_12_RIGID/RConn2 -- Revolute2/RConn1
  Planar2/RConn1 -- Right_Femur_3_RIGID/RConn3
  Cylindrical2/LConn1 -- x0_625_bearring_9_RIGID/RConn1
  Cylindrical2/RConn1 -- Right_Femur_3_RIGID/RConn2
  Revolute13/LConn1 -- Right_Femur_3_RIGID/RConn1
  Revolute13/RConn1 -- x0_625_bearring_17_RIGID/LConn1
  Cover_Thorax_1_RIGID/RConn1 -- Planar3/LConn1
  Planar3/RConn1 -- Thorax_1_RIGID/LConn3
  Planar4/LConn1 -- Thorax_1_RIGID/RConn2
  Planar4/RConn1 -- x0_625_bearring_2_RIGID/RConn1
  DS3218MG_v1_2_RIGID/LConn1 -- Thorax_1_RIGID/LConn2
  DS3218MG_v1_12_RIGID/RConn1 -- Parallel/LConn1
  DS3218MG_v1_3_RIGID/LConn1 -- Thorax_1_RIGID/RConn4
  Battery_bank_1_RIGID/LConn1 -- battery_cover_1_RIGID/LConn2
  Abdomen_1_RIGID/LConn8 -- battery_cover_1_RIGID/LConn1
  Coxa_12_RIGID/LConn1 -- Coxa_2_RIGID/RConn1
  DS3218MG_v1_3_RIGID/RConn1 -- Revolute14/LConn1
  Coxa_2_RIGID/LConn1 -- Revolute14/RConn1
  Coxa_13_RIGID/LConn1 -- Coxa_3_RIGID/RConn1
  DS3218MG_v1_5_RIGID/RConn1 -- Revolute15/LConn1
  Coxa_3_RIGID/LConn1 -- Revolute15/RConn1
  Coxa_4_RIGID/LConn1 -- Coxa_8_RIGID/RConn2
  Left_Femur_3_RIGID/RConn2 -- Parallel/RConn1
  DS3218MG_v1_4_RIGID/RConn1 -- Revolute16/LConn1
  Coxa_4_RIGID/RConn1 -- Revolute16/RConn1
  Coxa_5_RIGID/LConn2 -- Coxa_9_RIGID/RConn2
  DS3218MG_v1_1_RIGID/LConn1 -- Revolute17/LConn1
  Coxa_5_RIGID/LConn1 -- Revolute17/RConn1
  Coxa_10_RIGID/RConn1 -- Coxa_6_RIGID/LConn2
  DS3218MG_v1_6_RIGID/RConn1 -- Revolute18/LConn1
  Coxa_6_RIGID/LConn1 -- Revolute18/RConn1
  Coxa_11_RIGID/LConn2 -- Coxa_7_RIGID/LConn1
  DS3218MG_v1_2_RIGID/RConn1 -- Revolute19/LConn1
  Coxa_13_RIGID/RConn2 -- Revolute3/LConn1
  Coxa_7_RIGID/RConn1 -- Revolute19/RConn1
  Coxa_8_RIGID/LConn1 -- Revolute20/LConn1
  Revolute20/RConn1 -- x0_625_bearring_7_RIGID/LConn2
  Coxa_8_RIGID/LConn2 -- Planar5/LConn1
  Left_Femur_3_RIGID/RConn3 -- Planar5/RConn1
  Coxa_9_RIGID/RConn1 -- Revolute21/LConn1
  Revolute21/RConn1 -- x0_625_bearring_9_RIGID/RConn2
  DS3218MG_v1_2_RIGID/RConn2 -- Prismatic/LConn1
  Cover_Thorax_1_RIGID/LConn1 -- Prismatic/RConn1
  Pan_component_1_RIGID/RConn2 -- Revolute22/LConn1
